simulink model "power_estimate_calibration"  (Simulink 6.6)
settings: Solver=FixedStepDiscrete  StartTime=0.0  StopTime=inf  FixedStep=parameters.model.sample_time  RelTol=1e-3
values from neighbouring files (symbols this model uses):
  cad_ref = 20    [power_est_20rpm.mat]    (also in power_est_20rpm_2_cadence.mat; power_est_40rpm.mat = 40; power_est_70rpm.mat = 70; power_est_cadence_nomotor.mat = 40)
  freq_range = 865.41    [power_est_20rpm.mat]    (also in power_est_20rpm_2_cadence.mat; power_est_40rpm.mat; power_est_70rpm.mat; power_est_cadence_nomotor.mat)
  freq_zero = 39.49    [power_est_20rpm.mat]    (also in power_est_20rpm_2_cadence.mat; power_est_40rpm.mat; power_est_70rpm.mat; power_est_cadence_nomotor.mat)
  parameters =     [power_est_20rpm.mat]    (also in power_est_20rpm_2_cadence.mat; power_est_40rpm.mat; power_est_70rpm.mat; power_est_cadence_nomotor.mat)
  phio_mat = [1 -0.559 0.0775]    [power_est_20rpm.mat]    (also in power_est_20rpm_2_cadence.mat; power_est_40rpm.mat; power_est_70rpm.mat; power_est_cadence_nomotor.mat)
  Pi = 0    [power_est_20rpm.mat]    (also in power_est_20rpm_2_cadence.mat; power_est_40rpm.mat; power_est_70rpm.mat; power_est_cadence_nomotor.mat)
  Pw = -5    [power_est_20rpm.mat]    (also in power_est_20rpm_2_cadence.mat; power_est_40rpm.mat; power_est_70rpm.mat; power_est_cadence_nomotor.mat = 0)
  ro_mat = [0.7602 -0.2976 0.0591]    [power_est_20rpm.mat]    (also in power_est_20rpm_2_cadence.mat; power_est_40rpm.mat; power_est_70rpm.mat; power_est_cadence_nomotor.mat)
  s_mat = [0.0005025 -0.0003467]    [power_est_20rpm.mat]    (also in power_est_20rpm_2_cadence.mat; power_est_40rpm.mat; power_est_70rpm.mat; power_est_cadence_nomotor.mat)
  slope = 14.1374    [power_est_20rpm.mat]    (also in power_est_20rpm_2_cadence.mat; power_est_40rpm.mat; power_est_70rpm.mat; power_est_cadence_nomotor.mat)
  stim_max = 0    [power_est_20rpm.mat]    (also in power_est_20rpm_2_cadence.mat; power_est_40rpm.mat; power_est_70rpm.mat; power_est_cadence_nomotor.mat)
  stim_min = 0    [power_est_20rpm.mat]    (also in power_est_20rpm_2_cadence.mat; power_est_40rpm.mat; power_est_70rpm.mat; power_est_cadence_nomotor.mat)
  t_mat = [0.0002987 -0.000166 2.31e-05]    [power_est_20rpm.mat]    (also in power_est_20rpm_2_cadence.mat; power_est_40rpm.mat; power_est_70rpm.mat; power_est_cadence_nomotor.mat)
  Ti = 6000    [power_est_20rpm.mat]    (also in power_est_20rpm_2_cadence.mat; power_est_40rpm.mat; power_est_70rpm.mat; power_est_cadence_nomotor.mat)
  Ts = 20    [power_est_20rpm.mat]    (also in power_est_20rpm_2_cadence.mat; power_est_40rpm.mat; power_est_70rpm.mat; power_est_cadence_nomotor.mat)
  Tw = 6000    [power_est_20rpm.mat]    (also in power_est_20rpm_2_cadence.mat; power_est_40rpm.mat; power_est_70rpm.mat; power_est_cadence_nomotor.mat)
libraries: simulink x3, ni_lib x2, Stimulation_Currents_lib x1, stimulation_staticAngles_lib x1
(part 2 of 2)

== system power_estimate_calibration/Stimulation_System/Serial_Stimulation_System/Stimulation Activation/Angle Check1/0 < stop < 360 ==
  In1 : Inport
  Gain : Gain  Gain=360  SaturateOnIntegerOverflow=on
  Gain1 : Gain  Gain=1/360  SaturateOnIntegerOverflow=on
  Rounding Function : Rounding
  Sum : Sum  Inputs=|+-  SaturateOnIntegerOverflow=on  InputSameDT=on
  Out1 : Outport
  wires:
  Sum/1 -> Out1/1
  Gain/1 -> Sum/2
  Rounding Function/1 -> Gain/1
  Gain1/1 -> Rounding Function/1
  In1/1 -> Gain1/1, Sum/1
